simulink model "Non_Linear_Model_Inverted_Pendulum"  (R2022a)
settings: Solver=VariableStepAuto  StartTime=0.0  StopTime=10.0  RelTol=1e-3
values from neighbouring files (symbols this model uses):
  b = 0.00007892    (= 7.892e-05)    [Init_Setup_LQRArd.m]    (also in Parameters.m = 7.892e-06; Sim_Inverted_Pendulum.m = 1)
  c = 0.63    [Init_Setup_LQRArd.m]    (also in Parameters.m = 20)
  g = 9.81    [Init_Setup_LQRArd.m]    (also in Parameters.m; Sim_Inverted_Pendulum.m = -10; lqr_cartpend.m = -10; poleplace_cartpend.m = -10)
  I = 0.022    [Init_Setup_LQRArd.m]    (also in Parameters.m = 0.0025)
  L = 2    [Sim_Inverted_Pendulum.m]    (also in lqr_cartpend.m; poleplace_cartpend.m)
  m = 0.166    [Init_Setup_LQRArd.m]    (also in Parameters.m = 0.038; Sim_Inverted_Pendulum.m = 1; lqr_cartpend.m = 1; poleplace_cartpend.m = 1)
  M = 0.2    [Init_Setup_LQRArd.m]    (also in Parameters.m; Sim_Inverted_Pendulum.m = 5; lqr_cartpend.m = 5; poleplace_cartpend.m = 5)
settings Model: Creator=sokse  LastModifiedBy=sokse

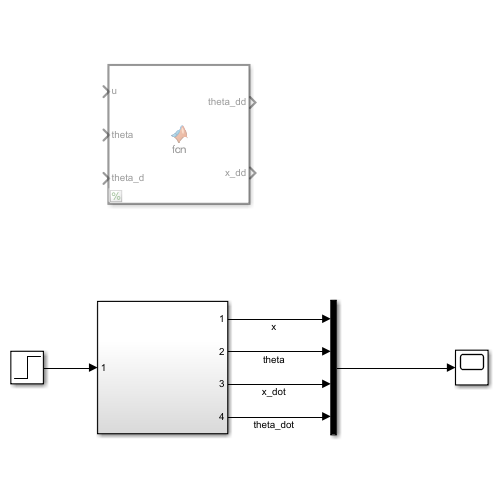
[thumbnail: Simulink's stored preview of the top-level diagram]
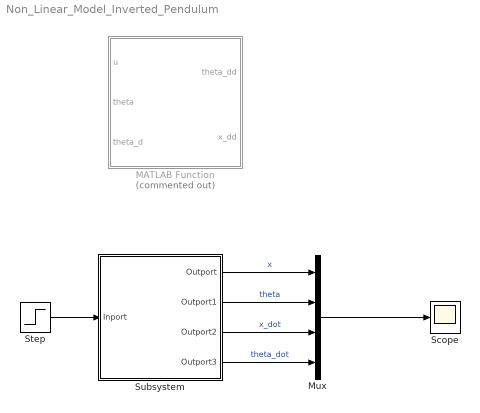
== system Non_Linear_Model_Inverted_Pendulum ==
  MATLAB Function : MATLAB Function  Commented=on  TreatAsAtomicUnit=on
  Mux : Mux
  Scope : Scope
  Step : Step  SampleTime=0
  Subsystem : Subsystem
  wires:
  Step/1 -> Subsystem/1(Inport)
  Subsystem/1(Outport) -> Mux/1  "x"
  Subsystem/2(Outport1) -> Mux/2  "theta"
  Subsystem/3(Outport2) -> Mux/3  "x_dot"
  Subsystem/4(Outport3) -> Mux/4  "theta_dot"
  Mux/1 -> Scope/1

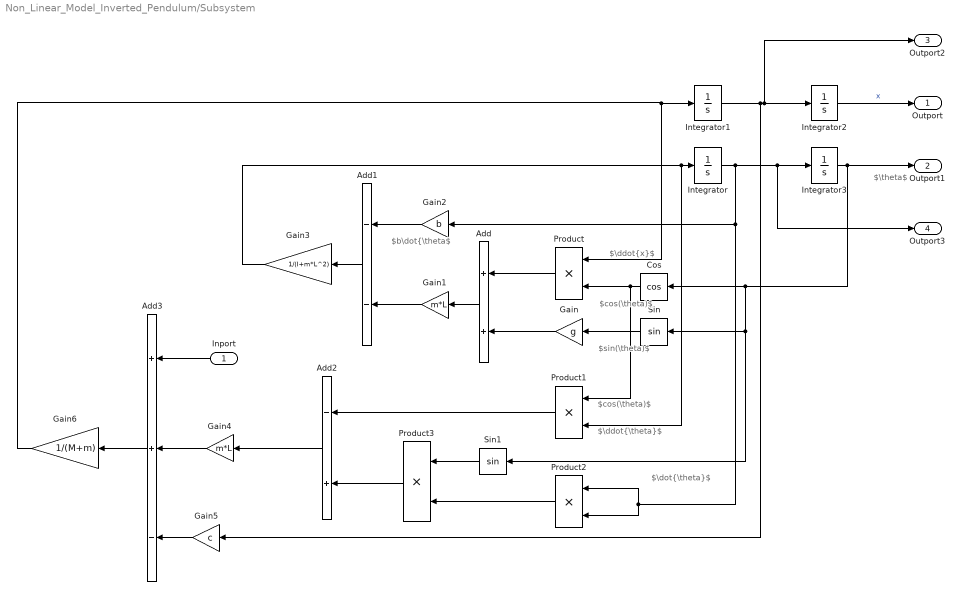
== system Non_Linear_Model_Inverted_Pendulum/Subsystem ==
  note: $cos(\theta)$
  note: $\theta$
  note: $\ddot{x}$
  note: $sin(\theta)$
  note: $b\dot{\theta$
  note: $cos(\theta)$
  note: $\ddot{\theta}$
  note: $\dot{\theta}$
  Inport : Inport
  Add : Sum
  Add1 : Sum  Inputs=--
  Add2 : Sum  Inputs=-+
  Add3 : Sum  Inputs=++-
  Cos : Trigonometry  Operator=cos
  Gain : Gain  Gain=g
  Gain1 : Gain  Gain=m*L
  Gain2 : Gain  Gain=b
  Gain3 : Gain  Gain=1/(I+m*L^2)
  Gain4 : Gain  Gain=m*L
  Gain5 : Gain  Gain=c
  Gain6 : Gain  Gain=1/(M+m)
  Integrator{,1..3} (4 alike) : Integrator
  Product{,1..3} (4 alike) : Product
  Sin : Trigonometry
  Sin1 : Trigonometry
  Outport : Outport
  Outport1 : Outport  Port=2
  Outport2 : Outport  Port=3
  Outport3 : Outport  Port=4
  wires:
  Integrator3/1 -> Outport1/1, Sin/1, Sin1/1, Cos/1
  Gain4/1 -> Add3/2
  Add/1 -> Gain1/1
  Add2/1 -> Gain4/1
  Cos/1 -> Product1/1, Product/2
  Gain1/1 -> Add1/2
  Gain6/1 -> Product/1, Integrator1/1
  Gain2/1 -> Add1/1
  Gain5/1 -> Add3/3
  Product2/1 -> Product3/2
  Integrator/1 -> Product2/1, Product2/2, Gain2/1, Outport3/1, Integrator3/1
  Product/1 -> Add/1
  Integrator1/1 -> Gain5/1, Outport2/1, Integrator2/1
  Product1/1 -> Add2/1
  Gain3/1 -> Product1/2, Integrator/1
  Add1/1 -> Gain3/1
  Sin1/1 -> Product3/1
  Integrator2/1 -> Outport/1  "x"
  Add3/1 -> Gain6/1
  Gain/1 -> Add/2
  Inport/1 -> Add3/1
  Product3/1 -> Add2/2
  Sin/1 -> Gain/1

== matlab function Non_Linear_Model_Inverted_Pendulum/MATLAB Function ==
  data: u input; theta_dd output; theta input; theta_d input; x_dd output
function [theta_dd, x_dd] = fcn(u,theta,theta_d )


theta_dd = 1/I+m*l^2*((x_dd*cos(theta)+g*sin(theta))*m*l - b*theta_d); 
x_dd = 1/(M+m)*((-theta_dd*cos(theta)+theta_d^2*sin(theta))*m*l-c*x_d+u);
